simulink model "flow"  (R2014a)
settings: Solver=FixedStepDiscrete  StartTime=0.0  StopTime=10  FixedStep=0.1  RelTol=1e-3
settings Model: Creator=lenovo  LastModifiedBy=DELL
settings SolverCC: AutoInsertRateTranBlk=on
settings DataIOCC: SaveFormat=StructureWithTime
settings DebuggingCC: MergeDetectMultiDrivingBlocksExec=error  SolverPrmCheckMsg=none  FrameProcessingCompatibilityMsg=error
settings HardwareCC: ProdBitPerPointer=64  ProdLargestAtomicFloat=Float  ProdIntDivRoundTo=Zero  ProdEndianess=LittleEndian  ProdHWDeviceType=Specified
settings ModelReferenceCC: PropagateSignalLabelsOutOfModel=on

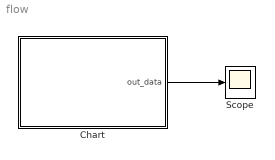
== system flow ==
  Chart : Stateflow chart  TreatAsAtomicUnit=on
      settings: PermitHierarchicalResolution=ParametersOnly
  Scope : Scope
      settings: TimeRange=auto  MaxDataPoints=5000  SaveToWorkspace=off  SaveName=ScopeData  YMin=-18.75  YMax=168.75  SampleTime=-1
  wires:
  Chart/1(out_data) -> Scope/1

== stateflow chart flow/Chart ==
  state A
  state B
    (default) -> (junction 10) : {i=1;}
    (junction 10) -> (junction 12) [order 1] : [i<=3]
    (junction 13) -> (junction 10) : {i = i + 1;}
    (junction 10) -> (junction 14) [order 2]
    (junction 12) -> (junction 13) : {out_data(i)=out_data(i)+i;}
  (default) -> A
  A -> B
  B -> A
  data: out_data output =[0,0,0]; i local
